simulink model "TerminatingJunction_2018a"  (R2018a)
settings: Solver=VariableStepAuto  StartTime=0.0  StopTime=10.0  RelTol=1e-3
settings Model: Creator=apple  LastModifiedBy=apple
settings DataIOCC: ReturnWorkspaceOutputs=on
settings SFSimCC: SimUseLocalCustomCode=on
settings RTWCC: RTWUseLocalCustomCode=on

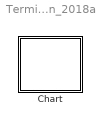
== system TerminatingJunction_2018a ==
  Chart : Stateflow chart  TreatAsAtomicUnit=on

== stateflow chart TerminatingJunction_2018a/Chart ==
  state A
    en:fprintf("Entry A");
    du:fprintf("During A");
    ex:fprintf("Exit A");
  state B
    en:fprintf("Entry B");
    du:fprintf("During B");
    ex:fprintf("Exit B");
  (default) -> A : {x = 0;}
  A -> (junction 1) [order 1] : [x > -1]{fprintf("Condition Action1");}
  (junction 1) -> (junction 7) [order 1] : [x > -1]{fprintf("Condition Action3");}
  (junction 7) -> B [order 1] : [x > 0]{fprintf("Condition Action4");}
  A -> (junction 1) [order 2] : [x > -3]{fprintf("Condition Action2");}
  (junction 1) -> (junction 10) [order 2]
  (junction 7) -> (junction 12) [order 2]
